simulink model "TTS2_EXT"  (R2024b)
settings: Solver=FixedStepAuto  StartTime=0.0  StopTime=inf  FixedStep=0.01  RelTol=1e-3
model workspace (MAT data in the model file):
  amp_f1 = -100
  amp_f10 = 0.5
  amp_f11 = -0.1
  amp_f12 = 1
  amp_f13 = 0.5
  amp_f14 = -20
  amp_f15 = 0.5
  amp_f16 = 0.5
  amp_f17 = 20
  amp_f18 = -30
  amp_f19 = 0.1
  amp_f2 = -20
  amp_f20 = -20
  amp_f21 = 20
  amp_f3 = -30
  amp_f4 = -30
  amp_f5 = -10
  amp_f51 = -10
  amp_f52 = -30
  amp_f53 = -30
  amp_f54 = 20
  amp_f55 = -100
  amp_f6 = -30
  amp_f7 = -30
  amp_f8 = -30
  amp_f9 = 1
  from_f1 = 570
  from_f10 = 5970
  from_f11 = 6570
  from_f12 = 7170
  from_f13 = 7770
  from_f14 = 8370
  from_f15 = 8970
  from_f16 = 9570
  from_f17 = 10170
  from_f18 = 10770
  from_f19 = 11370
  from_f2 = 1170
  from_f20 = 11970
  from_f21 = 12570
  from_f3 = 1770
  from_f4 = 2370
  from_f5 = 2970
  from_f51 = 13170
  from_f52 = 13770
  from_f53 = 14370
  from_f54 = 14970
  from_f55 = 15570
  from_f6 = 3570
  from_f7 = 4170
  from_f8 = 4770
  from_f9 = 5370
libraries: simulink x52, lab310_library x26, opclib x3
(part 2 of 3)

== system TTS2_EXT/PID/Antiwindup ==
  CV : Inport
  Logical Operator : Logic  Operator=NOR  AllPortsSameDT=off  OutDataTypeStr=boolean
  Relational Operator : RelationalOperator  Operator=<=  OutDataTypeStr=boolean  RndMeth=Simplest  InputSameDT=off
  Relational Operator1 : RelationalOperator  OutDataTypeStr=boolean  RndMeth=Simplest  InputSameDT=off
  norm CV max : Constant
  norm CVmin : Constant  Value=0
  enable : Outport  VectorParamsAs1DForOutWhenUnconnected=off
  wires:
  norm CVmin/1 -> Relational Operator/2
  norm CV max/1 -> Relational Operator1/2
  CV/1 -> Relational Operator1/1, Relational Operator/1
  Relational Operator/1 -> Logical Operator/1
  Relational Operator1/1 -> Logical Operator/2
  Logical Operator/1 -> enable/1

== system TTS2_EXT/TTS2/Disturbance ==
  Control : Inport
  Add : Sum  Inputs=2
  Add1 : Sum  Inputs=2
  Bus Selector : BusSelector  OutputSignals=PrDistValue,PrDistShift,EnPrDistShift,EnPrDist
  Product : Product
  Pulse Generator : DiscretePulseGenerator  PulseType=Time based  Period=480  PulseWidth=25
  Pulse Generator1 : DiscretePulseGenerator  PulseType=Time based  Amplitude=-1  Period=480  PulseWidth=25  PhaseDelay=240
  Switch : Switch  Criteria=u2 > Threshold  Threshold=0.5  SaturateOnIntegerOverflow=off
  Switch1 : Switch  Criteria=u2 > Threshold  Threshold=0.5  SaturateOnIntegerOverflow=off  InputSameDT=off
  no dist shift : Constant  Value=0
  dist[%] : Outport  VectorParamsAs1DForOutWhenUnconnected=off
  wires:
  Control/1 -> Bus Selector/1
  Bus Selector/2 -> Switch1/1  "<PrDistShift>"
  Bus Selector/3 -> Switch1/2  "<EnPrDistShift>"
  Switch/1 -> dist[%]/1  "PrShift+Dist"
  Switch1/1 -> Switch/3, Add/2
  Bus Selector/4 -> Switch/2  "<EnPrDist>"
  no dist shift/1 -> Switch1/3
  Add/1 -> Switch/1
  Pulse Generator/1 -> Add1/1
  Pulse Generator1/1 -> Add1/2
  Bus Selector/1 -> Product/2  "<PrDistValue>"
  Product/1 -> Add/1
  Add1/1 -> Product/1

== system TTS2_EXT/TTS2/Disturbance: Pump+pipe+control valve ==
  CV : Inport
  Patm[kPa] : Constant  Value=1.013  OutMin=[0.1013]  OutMax=[2.026]
  Pump control [%] : Constant  Value=pc  mask{pc=100.0}
      mask prompts: pc "Pump control"
  Pump+Pipe : Subsystem
  VB : Subsystem
  F[m3/h] : Outport  VectorParamsAs1DForOutWhenUnconnected=off
  wires:
  Pump+Pipe/1(P[kPa]) -> VB/2(P1[kPa])
  CV/1 -> VB/1(CV[%])
  Patm[kPa]/1 -> VB/3(P2[kPa])
  VB/1(F[m3/h]) -> Pump+Pipe/2(F[m3/h]), F[m3/h]/1
  Pump control [%]/1 -> Pump+Pipe/1(MP)

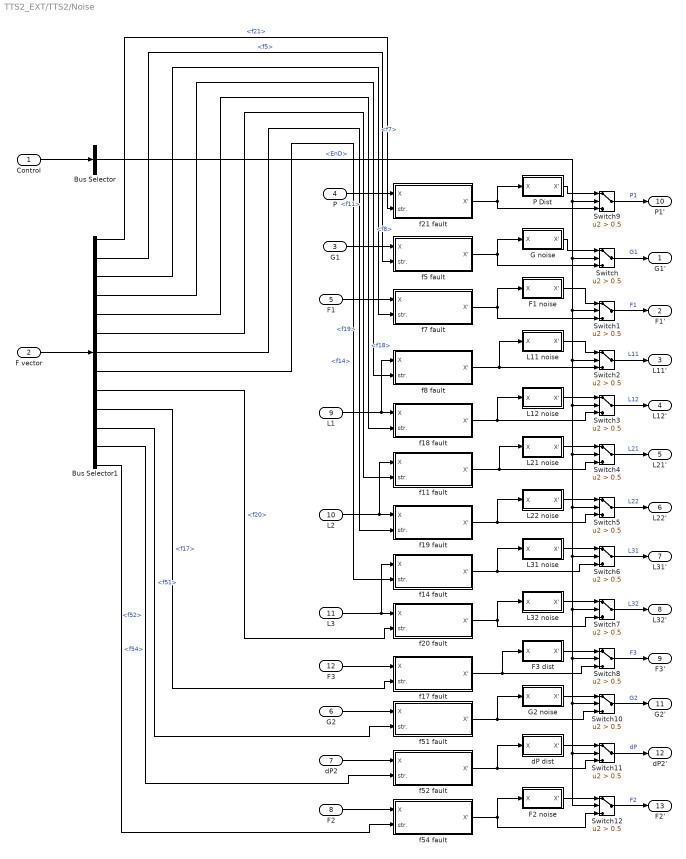
== system TTS2_EXT/TTS2/Noise ==
  Control : Inport
  F vector : Inport  Port=2
  G1 : Inport  Port=3
  P : Inport  Port=4
  F1 : Inport  Port=5
  G2 : Inport  Port=6
  dP2 : Inport  Port=7
  F2 : Inport  Port=8
  L1 : Inport  Port=9
  L2 : Inport  Port=10
  L3 : Inport  Port=11
  F3 : Inport  Port=12
  Bus Selector : BusSelector  OutputSignals=EnD
  Bus Selector1 : BusSelector  OutputSignals=f21,f5,f7,f8,f18,f11,f19,f14,f20,f17,f51,f52,f54
  F1 noise : Subsystem
  F2 noise : Subsystem
  F3 dist : Subsystem
  G noise : Subsystem
  G2 noise : Subsystem
  L11 noise : Subsystem
  L12 noise : Subsystem
  L21 noise : Subsystem
  L22 noise : Subsystem
  L31 noise : Subsystem
  L32 noise : Subsystem
  P Dist : Subsystem
  Switch{,1..12} (13 alike) : Switch  Criteria=u2 > Threshold  Threshold=0.5  SaturateOnIntegerOverflow=off  InputSameDT=off
  dP dist : Subsystem
  f11 fault : Subsystem
  f14 fault : Subsystem
  f17 fault : Subsystem
  f18 fault : Subsystem
  f19 fault : Subsystem
  f20 fault : Subsystem
  f21 fault : Subsystem
  f5 fault : Subsystem
  f51 fault : Subsystem
  f52 fault : Subsystem
  f54 fault : Subsystem
  f7 fault : Subsystem
  f8 fault : Subsystem
  G1' : Outport  VectorParamsAs1DForOutWhenUnconnected=off
  F1' : Outport  Port=2  VectorParamsAs1DForOutWhenUnconnected=off
  L11' : Outport  Port=3  VectorParamsAs1DForOutWhenUnconnected=off
  L12' : Outport  Port=4  VectorParamsAs1DForOutWhenUnconnected=off
  L21' : Outport  Port=5  VectorParamsAs1DForOutWhenUnconnected=off
  L22' : Outport  Port=6  VectorParamsAs1DForOutWhenUnconnected=off
  L31' : Outport  Port=7  VectorParamsAs1DForOutWhenUnconnected=off
  L32' : Outport  Port=8  VectorParamsAs1DForOutWhenUnconnected=off
  F3' : Outport  Port=9  VectorParamsAs1DForOutWhenUnconnected=off
  P1' : Outport  Port=10  VectorParamsAs1DForOutWhenUnconnected=off
  G2' : Outport  Port=11  VectorParamsAs1DForOutWhenUnconnected=off
  dP2' : Outport  Port=12  VectorParamsAs1DForOutWhenUnconnected=off
  F2' : Outport  Port=13  VectorParamsAs1DForOutWhenUnconnected=off
  wires:
  f21 fault/1(X') -> P Dist/1(X), Switch9/3
  P Dist/1(X') -> Switch9/1
  Switch9/1 -> P1'/1  "P1"
  P/1 -> f21 fault/1(X)
  Switch2/1 -> L11'/1  "L11"
  Switch8/1 -> F3'/1  "F3"
  Switch7/1 -> L32'/1  "L32"
  F1 noise/1(X') -> Switch1/1
  Switch3/1 -> L12'/1  "L12"
  Switch4/1 -> L21'/1  "L21"
  Switch6/1 -> L31'/1  "L31"
  L11 noise/1(X') -> Switch2/1
  G noise/1(X') -> Switch/1
  Switch5/1 -> L22'/1  "L22"
  f20 fault/1(X') -> Switch7/3, L32 noise/1(X)
  F3 dist/1(X') -> Switch8/1
  f11 fault/1(X') -> Switch4/3, L21 noise/1(X)
  L32 noise/1(X') -> Switch7/1
  L31 noise/1(X') -> Switch6/1
  f18 fault/1(X') -> Switch3/3, L12 noise/1(X)
  F1/1 -> f7 fault/1(X)
  L22 noise/1(X') -> Switch5/1
  L1/1 -> f18 fault/1(X), f8 fault/1(X)
  L2/1 -> f11 fault/1(X), f19 fault/1(X)
  Switch/1 -> G1'/1  "G1"
  f5 fault/1(X') -> Switch/3, G noise/1(X)
  L21 noise/1(X') -> Switch4/1
  f19 fault/1(X') -> Switch5/3, L22 noise/1(X)
  Bus Selector/1 -> Switch9/2, Switch8/2, Switch12/2, Switch11/2, Switch10/2, Switch7/2, Switch6/2, Switch5/2, Switch4/2, Switch3/2, Switch2/2, Switch1/2, Switch/2  "<EnD>"
  f17 fault/1(X') -> F3 dist/1(X), Switch8/3
  Switch1/1 -> F1'/1  "F1"
  L12 noise/1(X') -> Switch3/1
  f8 fault/1(X') -> Switch2/3, L11 noise/1(X)
  f14 fault/1(X') -> Switch6/3, L31 noise/1(X)
  f7 fault/1(X') -> Switch1/3, F1 noise/1(X)
  L3/1 -> f14 fault/1(X), f20 fault/1(X)
  G1/1 -> f5 fault/1(X)
  Control/1 -> Bus Selector/1
  F vector/1 -> Bus Selector1/1
  Bus Selector1/1 -> f21 fault/2(str.)  "<f21>"
  Bus Selector1/2 -> f5 fault/2(str.)  "<f5>"
  Bus Selector1/3 -> f7 fault/2(str.)  "<f7>"
  Bus Selector1/4 -> f8 fault/2(str.)  "<f8>"
  Bus Selector1/5 -> f18 fault/2(str.)  "<f18>"
  Bus Selector1/6 -> f11 fault/2(str.)  "<f11>"
  Bus Selector1/7 -> f19 fault/2(str.)  "<f19>"
  Bus Selector1/8 -> f14 fault/2(str.)  "<f14>"
  Bus Selector1/9 -> f20 fault/2(str.)  "<f20>"
  Bus Selector1/10 -> f17 fault/2(str.)  "<f17>"
  dP2/1 -> f52 fault/1(X)
  G2/1 -> f51 fault/1(X)
  Switch12/1 -> F2'/1  "F2"
  Switch11/1 -> dP2'/1  "dP"
  Switch10/1 -> G2'/1  "G2"
  f54 fault/1(X') -> F2 noise/1(X), Switch12/3
  f52 fault/1(X') -> Switch11/3, dP dist/1(X)
  f51 fault/1(X') -> Switch10/3, G2 noise/1(X)
  G2 noise/1(X') -> Switch10/1
  dP dist/1(X') -> Switch11/1
  F2 noise/1(X') -> Switch12/1
  Bus Selector1/11 -> f51 fault/2(str.)  "<f51>"
  Bus Selector1/12 -> f52 fault/2(str.)  "<f52>"
  Bus Selector1/13 -> f54 fault/2(str.)  "<f54>"
  F2/1 -> f54 fault/1(X)
  F3/1 -> f17 fault/1(X)

== system TTS2_EXT/TTS2/Pump+pipe+control valve ==
  CV1 : Inport
  F vec : Inport  Port=2
  CV2 : Inport  Port=3
  Add : Sum
  Bus Selector : BusSelector  OutputSignals=f1,f2,f4,f6,f53
  Patm[kPa] : Constant  Value=1.013  OutMin=[0.1013]  OutMax=[2.026]
  Pump control [%] : Constant  Value=pc  mask{pc=100.0}
      mask prompts: pc "Pump control"
  Pump+Pipe : Subsystem
  V1 : Subsystem
  V2 : Subsystem
  f1 fault : Subsystem
  f2 fault : Subsystem
  X1[%] : Outport  VectorParamsAs1DForOutWhenUnconnected=off
  F1[m3/s] : Outport  Port=2  VectorParamsAs1DForOutWhenUnconnected=off
  dP1[kPa] : Outport  Port=3  VectorParamsAs1DForOutWhenUnconnected=off
  P[kPa] : Outport  Port=4  VectorParamsAs1DForOutWhenUnconnected=off
  X2[%] : Outport  Port=5  VectorParamsAs1DForOutWhenUnconnected=off
  F2[m3/s] : Outport  Port=6  VectorParamsAs1DForOutWhenUnconnected=off
  dP2[kPa] : Outport  Port=7  VectorParamsAs1DForOutWhenUnconnected=off
  wires:
  Pump control [%]/1 -> f1 fault/1(X)
  f2 fault/1(Xf) -> Pump+Pipe/1(MP)
  f1 fault/1(Xf) -> f2 fault/1(X)
  Bus Selector/2 -> f2 fault/2(str.)  "<f2>"
  Bus Selector/1 -> f1 fault/2(str.)  "<f1>"
  F vec/1 -> Bus Selector/1
  Pump+Pipe/1(P[kPa]) -> P[kPa]/1, V2/2(P1[kPa]), V1/2(P1[kPa])
  CV1/1 -> V1/1(CV[%])
  Patm[kPa]/1 -> V2/3(P2[kPa]), V1/3(P2[kPa])
  Bus Selector/3 -> V1/4(f04)  "<f4>"
  Bus Selector/4 -> V1/5(f06)  "<f6>"
  V1/1(X[%]) -> X1[%]/1
  V1/3(dP[kPa]) -> dP1[kPa]/1
  V1/2(F[m3/s]) -> Add/2, F1[m3/s]/1
  CV2/1 -> V2/1(CV[%])
  V2/1(X[%]) -> X2[%]/1
  V2/2(F[m3/s]) -> Add/1, F2[m3/s]/1
  V2/3(dP[kPa]) -> dP2[kPa]/1
  Bus Selector/5 -> V2/4(f53)  "<f53>"
  Add/1 -> Pump+Pipe/2(F[m3/h])

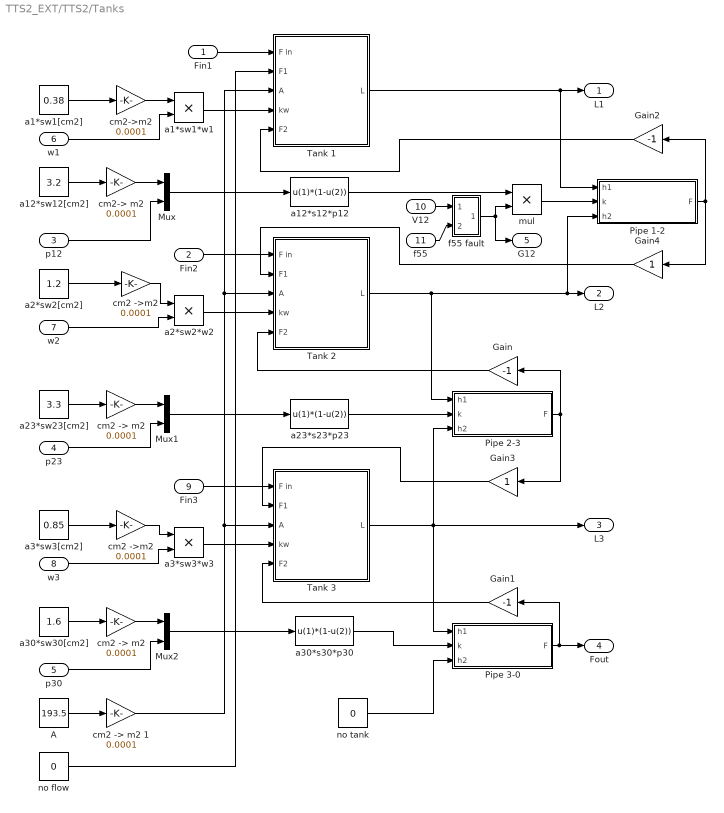
== system TTS2_EXT/TTS2/Tanks ==
  Fin1 : Inport
  Fin2 : Inport  Port=2
  p12 : Inport  Port=3
  p23 : Inport  Port=4
  p30 : Inport  Port=5
  w1 : Inport  Port=6
  w2 : Inport  Port=7
  w3 : Inport  Port=8
  Fin3 : Inport  Port=9
  V12 : Inport  Port=10
  f55 : Inport  Port=11
  A : Constant  Value=193.5
  Gain : Gain  Gain=-1
  Gain1 : Gain  Gain=-1
  Gain2 : Gain  Gain=-1
  Gain3 : Gain
  Gain4 : Gain
  Mux : Mux  Inputs=2
  Mux1 : Mux  Inputs=2
  Mux2 : Mux  Inputs=2
  Pipe 1-2 : Subsystem
  Pipe 2-3 : Subsystem
  Pipe 3-0 : Subsystem
  "Tank 1 " : Subsystem
  Tank 2 : Subsystem
  Tank 3 : Subsystem
  a1*sw1*w1 : Product
  a1*sw1[cm2] : Constant  Value=0.38
  a12*s12*p12 : Fcn  Expr=u(1)*(1-u(2))
  a12*sw12[cm2] : Constant  Value=3.2
  a2*sw2*w2 : Product
  a2*sw2[cm2] : Constant  Value=1.2
  a23*s23*p23 : Fcn  Expr=u(1)*(1-u(2))
  a23*sw23[cm2] : Constant  Value=3.3
  a3*sw3*w3 : Product
  a3*sw3[cm2] : Constant  Value=0.85
  a30*s30*p30 : Fcn  Expr=u(1)*(1-u(2))
  a30*sw30[cm2] : Constant  Value=1.6
  "cm2 -> m2" : Gain  Gain=0.0001
  "cm2 -> m2 " : Gain  Gain=0.0001
  "cm2 -> m2 1" : Gain  Gain=0.0001
  cm2 ->m2 : Gain  Gain=0.0001
  "cm2 ->m2 " : Gain  Gain=0.0001
  cm2-> m2 : Gain  Gain=0.0001
  cm2->m2 : Gain  Gain=0.0001
  f55 fault : Subsystem
  mul : Product
  no flow : Constant  Value=0
  no tank : Constant  Value=0
  L1 : Outport  VectorParamsAs1DForOutWhenUnconnected=off
  L2 : Outport  Port=2  VectorParamsAs1DForOutWhenUnconnected=off
  L3 : Outport  Port=3  VectorParamsAs1DForOutWhenUnconnected=off
  Fout : Outport  Port=4  VectorParamsAs1DForOutWhenUnconnected=off
  G12 : Outport  Port=5  VectorParamsAs1DForOutWhenUnconnected=off
  wires:
  Fin1/1 -> "Tank 1 "/1(F in)
  a1*sw1[cm2]/1 -> cm2->m2/1
  cm2->m2/1 -> a1*sw1*w1/1
  a1*sw1*w1/1 -> "Tank 1 "/4(kw)
  w1/1 -> a1*sw1*w1/2
  a12*sw12[cm2]/1 -> cm2-> m2/1
  cm2-> m2/1 -> Mux/1
  p12/1 -> Mux/2
  Mux/1 -> a12*s12*p12/1
  a2*sw2[cm2]/1 -> cm2 ->m2/1
  cm2 ->m2/1 -> a2*sw2*w2/1
  a23*sw23[cm2]/1 -> "cm2 -> m2"/1
  "cm2 -> m2"/1 -> Mux1/1
  Mux1/1 -> a23*s23*p23/1
  w2/1 -> a2*sw2*w2/2
  p23/1 -> Mux1/2
  a2*sw2*w2/1 -> Tank 2/4(kw)
  a3*sw3[cm2]/1 -> "cm2 ->m2 "/1
  "cm2 ->m2 "/1 -> a3*sw3*w3/1
  a30*sw30[cm2]/1 -> "cm2 -> m2 "/1
  "cm2 -> m2 "/1 -> Mux2/1
  w3/1 -> a3*sw3*w3/2
  p30/1 -> Mux2/2
  Mux2/1 -> a30*s30*p30/1
  a3*sw3*w3/1 -> Tank 3/4(kw)
  A/1 -> "cm2 -> m2 1"/1
  no flow/1 -> "Tank 1 "/2(F1)
  "cm2 -> m2 1"/1 -> Tank 3/3(A), Tank 2/3(A), "Tank 1 "/3(A)
  "Tank 1 "/1(L) -> Pipe 1-2/1(h1), L1/1
  a12*s12*p12/1 -> mul/1
  Tank 2/1(L) -> Pipe 1-2/3(h2), L2/1, Pipe 2-3/1(h1)
  a23*s23*p23/1 -> Pipe 2-3/2(k)
  Tank 3/1(L) -> Pipe 2-3/3(h2), Pipe 3-0/1(h1), L3/1
  a30*s30*p30/1 -> Pipe 3-0/2(k)
  no tank/1 -> Pipe 3-0/3(h2)
  Pipe 3-0/1(F) -> Fout/1, Gain1/1
  Pipe 2-3/1(F) -> Gain3/1, Gain/1
  Pipe 1-2/1(F) -> Gain2/1, Gain4/1
  Gain2/1 -> "Tank 1 "/5(F2)
  Gain/1 -> Tank 2/5(F2)
  Fin3/1 -> Tank 3/1(F in)
  Gain1/1 -> Tank 3/5(F2)
  Gain3/1 -> Tank 3/2(F1)
  Gain4/1 -> Tank 2/2(F1)
  Fin2/1 -> Tank 2/1(F in)
  mul/1 -> Pipe 1-2/2(k)
  V12/1 -> f55 fault/1(X)
  f55/1 -> f55 fault/2(str.)
  f55 fault/1(X') -> G12/1, mul/2

== system TTS2_EXT/TTS2/f3 fault ==
  X : Inport
  str. : Inport  Port=2
  Add : Sum
  Fcn : Fcn  Expr=u(1)*((u(2)/100)+1)
  Manual Switch : ManualSwitch  CurrentSetting=0
  Mux : Mux  Inputs=2
  X' : Outport  VectorParamsAs1DForOutWhenUnconnected=off
  wires:
  Mux/1 -> Fcn/1
  X/1 -> Add/1, Mux/1
  str./1 -> Add/2, Mux/2
  Manual Switch/1 -> X'/1
  Add/1 -> Manual Switch/1
  Fcn/1 -> Manual Switch/2

== system TTS2_EXT/Faults/f-control1/calc_f1 ==
  f-control : Inport
  f-s : Inport  Port=2
  Bus Selector : BusSelector  OutputSignals=EnF,AutoF
  Bus Selector1 : BusSelector  OutputSignals=f1
  Constant : Constant  Value=p
  Product : Product  Inputs=3
  Step : Step  Time=from  After=amp  SampleTime=0
  Step1 : Step  Time=from+st  After=-amp  SampleTime=0
  Subsystem : Subsystem
  Sum1 : Sum  Inputs=++|
  Switch:auto : Switch  Criteria=u2 > Threshold  Threshold=0.5  SaturateOnIntegerOverflow=off  InputSameDT=off
  f : Outport  VectorParamsAs1DForOutWhenUnconnected=off
  wires:
  f-control/1 -> Bus Selector/1
  f-s/1 -> Bus Selector1/1
  Product/1 -> f/1
  Bus Selector/1 -> Product/1  "<EnF>"
  Bus Selector/2 -> Switch:auto/2  "<AutoF>"
  Switch:auto/1 -> Product/2
  Step/1 -> Sum1/2
  Step1/1 -> Sum1/1
  Constant/1 -> Product/3
  Bus Selector1/1 -> Subsystem/1(w)  "<f1>"
  Subsystem/1(w_sim) -> Switch:auto/3
  Sum1/1 -> Switch:auto/1

== system TTS2_EXT/Faults/f-control1/calc_f10 ==
  f-control : Inport
  f-s : Inport  Port=2
  Bus Selector : BusSelector  OutputSignals=EnF,IncipF,AutoF
  Bus Selector1 : BusSelector  OutputSignals=f10
  Constant : Constant  Value=p
  Product : Product  Inputs=3
  RAMP : simulink/Sources/Ramp  slope=amp/st  start=from  InitialOutput=0
  Saturation : Saturate  UpperLimit=abs(amp)  LowerLimit=-abs(amp)
  Step : Step  Time=from  After=amp  SampleTime=0
  Step1 : Step  Time=from+st  After=-amp  SampleTime=0
  Subsystem : Subsystem
  Sum : Sum  Inputs=|++
  Sum1 : Sum  Inputs=++|
  Switch:auto : Switch  Criteria=u2 > Threshold  Threshold=0.5  SaturateOnIntegerOverflow=off  InputSameDT=off
  Switch:kind : Switch  Criteria=u2 > Threshold  Threshold=0.5  SaturateOnIntegerOverflow=off  InputSameDT=off
  f : Outport  VectorParamsAs1DForOutWhenUnconnected=off
  wires:
  f-control/1 -> Bus Selector/1
  f-s/1 -> Bus Selector1/1
  Product/1 -> f/1
  Bus Selector/1 -> Product/1  "<EnF>"
  Bus Selector/2 -> Subsystem/1(IncipF), Switch:kind/2  "<IncipF>"
  Bus Selector/3 -> Switch:auto/2  "<AutoF>"
  Switch:auto/1 -> Product/2
  Sum/1 -> Switch:kind/1
  Sum1/1 -> Switch:kind/3
  Switch:kind/1 -> Switch:auto/1
  Step/1 -> Sum1/2
  Step1/1 -> Sum/2, Sum1/1
  Saturation/1 -> Sum/1
  RAMP/1 -> Saturation/1
  Constant/1 -> Product/3
  Bus Selector1/1 -> Subsystem/2(w)  "<f10>"
  Subsystem/1(w_sim) -> Switch:auto/3

== system TTS2_EXT/Faults/f-control1/calc_f11 ==
  f-control : Inport
  f-s : Inport  Port=2
  Bus Selector : BusSelector  OutputSignals=EnF,IncipF,AutoF
  Bus Selector1 : BusSelector  OutputSignals=f11
  Constant : Constant  Value=p
  Product : Product  Inputs=3
  RAMP : simulink/Sources/Ramp  slope=amp/st  start=from  InitialOutput=0
  Saturation : Saturate  UpperLimit=abs(amp)  LowerLimit=-abs(amp)
  Step : Step  Time=from  After=amp  SampleTime=0
  Step1 : Step  Time=from+st  After=-amp  SampleTime=0
  Subsystem : Subsystem
  Sum : Sum  Inputs=|++
  Sum1 : Sum  Inputs=++|
  Switch:auto : Switch  Criteria=u2 > Threshold  Threshold=0.5  SaturateOnIntegerOverflow=off  InputSameDT=off
  Switch:kind : Switch  Criteria=u2 > Threshold  Threshold=0.5  SaturateOnIntegerOverflow=off  InputSameDT=off
  f : Outport  VectorParamsAs1DForOutWhenUnconnected=off
  wires:
  f-control/1 -> Bus Selector/1
  f-s/1 -> Bus Selector1/1
  Product/1 -> f/1
  Bus Selector/1 -> Product/1  "<EnF>"
  Bus Selector/2 -> Subsystem/1(IncipF), Switch:kind/2  "<IncipF>"
  Bus Selector/3 -> Switch:auto/2  "<AutoF>"
  Switch:auto/1 -> Product/2
  Sum/1 -> Switch:kind/1
  Sum1/1 -> Switch:kind/3
  Switch:kind/1 -> Switch:auto/1
  Step/1 -> Sum1/2
  Step1/1 -> Sum/2, Sum1/1
  Saturation/1 -> Sum/1
  RAMP/1 -> Saturation/1
  Constant/1 -> Product/3
  Bus Selector1/1 -> Subsystem/2(w)  "<f11>"
  Subsystem/1(w_sim) -> Switch:auto/3

== system TTS2_EXT/Faults/f-control1/calc_f12 ==
  f-control : Inport
  f-s : Inport  Port=2
  Bus Selector : BusSelector  OutputSignals=EnF,IncipF,AutoF
  Bus Selector1 : BusSelector  OutputSignals=f12
  Constant : Constant  Value=p
  Product : Product  Inputs=3
  RAMP : simulink/Sources/Ramp  slope=amp/st  start=from  InitialOutput=0
  Saturation : Saturate  UpperLimit=abs(amp)  LowerLimit=-abs(amp)
  Step : Step  Time=from  After=amp  SampleTime=0
  Step1 : Step  Time=from+st  After=-amp  SampleTime=0
  Subsystem : Subsystem
  Sum : Sum  Inputs=|++
  Sum1 : Sum  Inputs=++|
  Switch:auto : Switch  Criteria=u2 > Threshold  Threshold=0.5  SaturateOnIntegerOverflow=off  InputSameDT=off
  Switch:kind : Switch  Criteria=u2 > Threshold  Threshold=0.5  SaturateOnIntegerOverflow=off  InputSameDT=off
  f : Outport  VectorParamsAs1DForOutWhenUnconnected=off
  wires:
  f-control/1 -> Bus Selector/1
  f-s/1 -> Bus Selector1/1
  Product/1 -> f/1
  Bus Selector/1 -> Product/1  "<EnF>"
  Bus Selector/2 -> Subsystem/1(IncipF), Switch:kind/2  "<IncipF>"
  Bus Selector/3 -> Switch:auto/2  "<AutoF>"
  Switch:auto/1 -> Product/2
  Sum/1 -> Switch:kind/1
  Sum1/1 -> Switch:kind/3
  Switch:kind/1 -> Switch:auto/1
  Step/1 -> Sum1/2
  Step1/1 -> Sum/2, Sum1/1
  Saturation/1 -> Sum/1
  RAMP/1 -> Saturation/1
  Constant/1 -> Product/3
  Bus Selector1/1 -> Subsystem/2(w)  "<f12>"
  Subsystem/1(w_sim) -> Switch:auto/3

== system TTS2_EXT/Faults/f-control1/calc_f13 ==
  f-control : Inport
  f-s : Inport  Port=2
  Bus Selector : BusSelector  OutputSignals=EnF,IncipF,AutoF
  Bus Selector1 : BusSelector  OutputSignals=f13
  Constant : Constant  Value=p
  Product : Product  Inputs=3
  RAMP : simulink/Sources/Ramp  slope=amp/st  start=from  InitialOutput=0
  Saturation : Saturate  UpperLimit=abs(amp)  LowerLimit=-abs(amp)
  Step : Step  Time=from  After=amp  SampleTime=0
  Step1 : Step  Time=from+st  After=-amp  SampleTime=0
  Subsystem : Subsystem
  Sum : Sum  Inputs=|++
  Sum1 : Sum  Inputs=++|
  Switch:auto : Switch  Criteria=u2 > Threshold  Threshold=0.5  SaturateOnIntegerOverflow=off  InputSameDT=off
  Switch:kind : Switch  Criteria=u2 > Threshold  Threshold=0.5  SaturateOnIntegerOverflow=off  InputSameDT=off
  f : Outport  VectorParamsAs1DForOutWhenUnconnected=off
  wires:
  f-control/1 -> Bus Selector/1
  f-s/1 -> Bus Selector1/1
  Product/1 -> f/1
  Bus Selector/1 -> Product/1  "<EnF>"
  Bus Selector/2 -> Subsystem/1(IncipF), Switch:kind/2  "<IncipF>"
  Bus Selector/3 -> Switch:auto/2  "<AutoF>"
  Switch:auto/1 -> Product/2
  Sum/1 -> Switch:kind/1
  Sum1/1 -> Switch:kind/3
  Switch:kind/1 -> Switch:auto/1
  Step/1 -> Sum1/2
  Step1/1 -> Sum/2, Sum1/1
  Saturation/1 -> Sum/1
  RAMP/1 -> Saturation/1
  Constant/1 -> Product/3
  Bus Selector1/1 -> Subsystem/2(w)  "<f13>"
  Subsystem/1(w_sim) -> Switch:auto/3

== system TTS2_EXT/Faults/f-control1/calc_f14 ==
  f-control : Inport
  f-s : Inport  Port=2
  Bus Selector : BusSelector  OutputSignals=EnF,IncipF,AutoF
  Bus Selector1 : BusSelector  OutputSignals=f14
  Constant : Constant  Value=p
  Product : Product  Inputs=3
  RAMP : simulink/Sources/Ramp  slope=amp/st  start=from  InitialOutput=0
  Saturation : Saturate  UpperLimit=abs(amp)  LowerLimit=-abs(amp)
  Step : Step  Time=from  After=amp  SampleTime=0
  Step1 : Step  Time=from+st  After=-amp  SampleTime=0
  Subsystem : Subsystem
  Sum : Sum  Inputs=|++
  Sum1 : Sum  Inputs=++|
  Switch:auto : Switch  Criteria=u2 > Threshold  Threshold=0.5  SaturateOnIntegerOverflow=off  InputSameDT=off
  Switch:kind : Switch  Criteria=u2 > Threshold  Threshold=0.5  SaturateOnIntegerOverflow=off  InputSameDT=off
  f : Outport  VectorParamsAs1DForOutWhenUnconnected=off
  wires:
  f-control/1 -> Bus Selector/1
  f-s/1 -> Bus Selector1/1
  Product/1 -> f/1
  Bus Selector/1 -> Product/1  "<EnF>"
  Bus Selector/2 -> Subsystem/1(IncipF), Switch:kind/2  "<IncipF>"
  Bus Selector/3 -> Switch:auto/2  "<AutoF>"
  Switch:auto/1 -> Product/2
  Sum/1 -> Switch:kind/1
  Sum1/1 -> Switch:kind/3
  Switch:kind/1 -> Switch:auto/1
  Step/1 -> Sum1/2
  Step1/1 -> Sum/2, Sum1/1
  Saturation/1 -> Sum/1
  RAMP/1 -> Saturation/1
  Constant/1 -> Product/3
  Bus Selector1/1 -> Subsystem/2(w)  "<f14>"
  Subsystem/1(w_sim) -> Switch:auto/3

== system TTS2_EXT/Faults/f-control1/calc_f15 ==
  f-control : Inport
  f-s : Inport  Port=2
  Bus Selector : BusSelector  OutputSignals=EnF,IncipF,AutoF
  Bus Selector1 : BusSelector  OutputSignals=f15
  Constant : Constant  Value=p
  Product : Product  Inputs=3
  RAMP : simulink/Sources/Ramp  slope=amp/st  start=from  InitialOutput=0
  Saturation : Saturate  UpperLimit=abs(amp)  LowerLimit=-abs(amp)
  Step : Step  Time=from  After=amp  SampleTime=0
  Step1 : Step  Time=from+st  After=-amp  SampleTime=0
  Subsystem : Subsystem
  Sum : Sum  Inputs=|++
  Sum1 : Sum  Inputs=++|
  Switch:auto : Switch  Criteria=u2 > Threshold  Threshold=0.5  SaturateOnIntegerOverflow=off  InputSameDT=off
  Switch:kind : Switch  Criteria=u2 > Threshold  Threshold=0.5  SaturateOnIntegerOverflow=off  InputSameDT=off
  f : Outport  VectorParamsAs1DForOutWhenUnconnected=off
  wires:
  f-control/1 -> Bus Selector/1
  f-s/1 -> Bus Selector1/1
  Product/1 -> f/1
  Bus Selector/1 -> Product/1  "<EnF>"
  Bus Selector/2 -> Subsystem/1(IncipF), Switch:kind/2  "<IncipF>"
  Bus Selector/3 -> Switch:auto/2  "<AutoF>"
  Switch:auto/1 -> Product/2
  Sum/1 -> Switch:kind/1
  Sum1/1 -> Switch:kind/3
  Switch:kind/1 -> Switch:auto/1
  Step/1 -> Sum1/2
  Step1/1 -> Sum/2, Sum1/1
  Saturation/1 -> Sum/1
  RAMP/1 -> Saturation/1
  Constant/1 -> Product/3
  Bus Selector1/1 -> Subsystem/2(w)  "<f15>"
  Subsystem/1(w_sim) -> Switch:auto/3

== system TTS2_EXT/Faults/f-control1/calc_f16 ==
  f-control : Inport
  f-s : Inport  Port=2
  Bus Selector : BusSelector  OutputSignals=EnF,IncipF,AutoF
  Bus Selector1 : BusSelector  OutputSignals=f16
  Constant : Constant  Value=p
  Product : Product  Inputs=3
  RAMP : simulink/Sources/Ramp  slope=amp/st  start=from  InitialOutput=0
  Saturation : Saturate  UpperLimit=abs(amp)  LowerLimit=-abs(amp)
  Step : Step  Time=from  After=amp  SampleTime=0
  Step1 : Step  Time=from+st  After=-amp  SampleTime=0
  Subsystem : Subsystem
  Sum : Sum  Inputs=|++
  Sum1 : Sum  Inputs=++|
  Switch:auto : Switch  Criteria=u2 > Threshold  Threshold=0.5  SaturateOnIntegerOverflow=off  InputSameDT=off
  Switch:kind : Switch  Criteria=u2 > Threshold  Threshold=0.5  SaturateOnIntegerOverflow=off  InputSameDT=off
  f : Outport  VectorParamsAs1DForOutWhenUnconnected=off
  wires:
  f-control/1 -> Bus Selector/1
  f-s/1 -> Bus Selector1/1
  Product/1 -> f/1
  Bus Selector/1 -> Product/1  "<EnF>"
  Bus Selector/2 -> Subsystem/1(IncipF), Switch:kind/2  "<IncipF>"
  Bus Selector/3 -> Switch:auto/2  "<AutoF>"
  Switch:auto/1 -> Product/2
  Sum/1 -> Switch:kind/1
  Sum1/1 -> Switch:kind/3
  Switch:kind/1 -> Switch:auto/1
  Step/1 -> Sum1/2
  Step1/1 -> Sum/2, Sum1/1
  Saturation/1 -> Sum/1
  RAMP/1 -> Saturation/1
  Constant/1 -> Product/3
  Bus Selector1/1 -> Subsystem/2(w)  "<f16>"
  Subsystem/1(w_sim) -> Switch:auto/3

== system TTS2_EXT/Faults/f-control1/calc_f17 ==
  f-control : Inport
  f-s : Inport  Port=2
  Bus Selector : BusSelector  OutputSignals=EnF,IncipF,AutoF
  Bus Selector1 : BusSelector  OutputSignals=f17
  Constant : Constant  Value=p
  Product : Product  Inputs=3
  RAMP : simulink/Sources/Ramp  slope=amp/st  start=from  InitialOutput=0
  Saturation : Saturate  UpperLimit=abs(amp)  LowerLimit=-abs(amp)
  Step : Step  Time=from  After=amp  SampleTime=0
  Step1 : Step  Time=from+st  After=-amp  SampleTime=0
  Subsystem : Subsystem
  Sum : Sum  Inputs=|++
  Sum1 : Sum  Inputs=++|
  Switch:auto : Switch  Criteria=u2 > Threshold  Threshold=0.5  SaturateOnIntegerOverflow=off  InputSameDT=off
  Switch:kind : Switch  Criteria=u2 > Threshold  Threshold=0.5  SaturateOnIntegerOverflow=off  InputSameDT=off
  f : Outport  VectorParamsAs1DForOutWhenUnconnected=off
  wires:
  f-control/1 -> Bus Selector/1
  f-s/1 -> Bus Selector1/1
  Product/1 -> f/1
  Bus Selector/1 -> Product/1  "<EnF>"
  Bus Selector/2 -> Subsystem/1(IncipF), Switch:kind/2  "<IncipF>"
  Bus Selector/3 -> Switch:auto/2  "<AutoF>"
  Switch:auto/1 -> Product/2
  Sum/1 -> Switch:kind/1
  Sum1/1 -> Switch:kind/3
  Switch:kind/1 -> Switch:auto/1
  Step/1 -> Sum1/2
  Step1/1 -> Sum/2, Sum1/1
  Saturation/1 -> Sum/1
  RAMP/1 -> Saturation/1
  Constant/1 -> Product/3
  Bus Selector1/1 -> Subsystem/2(w)  "<f17>"
  Subsystem/1(w_sim) -> Switch:auto/3

== system TTS2_EXT/Faults/f-control1/calc_f18 ==
  f-control : Inport
  f-s : Inport  Port=2
  Bus Selector : BusSelector  OutputSignals=EnF,IncipF,AutoF
  Bus Selector1 : BusSelector  OutputSignals=f18
  Constant : Constant  Value=p
  Product : Product  Inputs=3
  RAMP : simulink/Sources/Ramp  slope=amp/st  start=from  InitialOutput=0
  Saturation : Saturate  UpperLimit=abs(amp)  LowerLimit=-abs(amp)
  Step : Step  Time=from  After=amp  SampleTime=0
  Step1 : Step  Time=from+st  After=-amp  SampleTime=0
  Subsystem : Subsystem
  Sum : Sum  Inputs=|++
  Sum1 : Sum  Inputs=++|
  Switch:auto : Switch  Criteria=u2 > Threshold  Threshold=0.5  SaturateOnIntegerOverflow=off  InputSameDT=off
  Switch:kind : Switch  Criteria=u2 > Threshold  Threshold=0.5  SaturateOnIntegerOverflow=off  InputSameDT=off
  f : Outport  VectorParamsAs1DForOutWhenUnconnected=off
  wires:
  f-control/1 -> Bus Selector/1
  f-s/1 -> Bus Selector1/1
  Product/1 -> f/1
  Bus Selector/1 -> Product/1  "<EnF>"
  Bus Selector/2 -> Subsystem/1(IncipF), Switch:kind/2  "<IncipF>"
  Bus Selector/3 -> Switch:auto/2  "<AutoF>"
  Switch:auto/1 -> Product/2
  Sum/1 -> Switch:kind/1
  Sum1/1 -> Switch:kind/3
  Switch:kind/1 -> Switch:auto/1
  Step/1 -> Sum1/2
  Step1/1 -> Sum/2, Sum1/1
  Saturation/1 -> Sum/1
  RAMP/1 -> Saturation/1
  Constant/1 -> Product/3
  Bus Selector1/1 -> Subsystem/2(w)  "<f18>"
  Subsystem/1(w_sim) -> Switch:auto/3

== system TTS2_EXT/Faults/f-control1/calc_f19 ==
  f-control : Inport
  f-s : Inport  Port=2
  Bus Selector : BusSelector  OutputSignals=EnF,IncipF,AutoF
  Bus Selector1 : BusSelector  OutputSignals=f19
  Constant : Constant  Value=p
  Product : Product  Inputs=3
  RAMP : simulink/Sources/Ramp  slope=amp/st  start=from  InitialOutput=0
  Saturation : Saturate  UpperLimit=abs(amp)  LowerLimit=-abs(amp)
  Step : Step  Time=from  After=amp  SampleTime=0
  Step1 : Step  Time=from+st  After=-amp  SampleTime=0
  Subsystem : Subsystem
  Sum : Sum  Inputs=|++
  Sum1 : Sum  Inputs=++|
  Switch:auto : Switch  Criteria=u2 > Threshold  Threshold=0.5  SaturateOnIntegerOverflow=off  InputSameDT=off
  Switch:kind : Switch  Criteria=u2 > Threshold  Threshold=0.5  SaturateOnIntegerOverflow=off  InputSameDT=off
  f : Outport  VectorParamsAs1DForOutWhenUnconnected=off
  wires:
  f-control/1 -> Bus Selector/1
  f-s/1 -> Bus Selector1/1
  Product/1 -> f/1
  Bus Selector/1 -> Product/1  "<EnF>"
  Bus Selector/2 -> Subsystem/1(IncipF), Switch:kind/2  "<IncipF>"
  Bus Selector/3 -> Switch:auto/2  "<AutoF>"
  Switch:auto/1 -> Product/2
  Sum/1 -> Switch:kind/1
  Sum1/1 -> Switch:kind/3
  Switch:kind/1 -> Switch:auto/1
  Step/1 -> Sum1/2
  Step1/1 -> Sum/2, Sum1/1
  Saturation/1 -> Sum/1
  RAMP/1 -> Saturation/1
  Constant/1 -> Product/3
  Bus Selector1/1 -> Subsystem/2(w)  "<f19>"
  Subsystem/1(w_sim) -> Switch:auto/3

== system TTS2_EXT/Faults/f-control1/calc_f2 ==
  f-control : Inport
  f-s : Inport  Port=2
  Bus Selector : BusSelector  OutputSignals=EnF,IncipF,AutoF
  Bus Selector1 : BusSelector  OutputSignals=f2
  Constant : Constant  Value=p
  Product : Product  Inputs=3
  RAMP : simulink/Sources/Ramp  slope=amp/st  start=from  InitialOutput=0
  Saturation : Saturate  UpperLimit=abs(amp)  LowerLimit=-abs(amp)
  Step : Step  Time=from  After=amp  SampleTime=0
  Step1 : Step  Time=from+st  After=-amp  SampleTime=0
  Subsystem : Subsystem
  Sum : Sum  Inputs=|++
  Sum1 : Sum  Inputs=++|
  Switch:auto : Switch  Criteria=u2 > Threshold  Threshold=0.5  SaturateOnIntegerOverflow=off  InputSameDT=off
  Switch:kind : Switch  Criteria=u2 > Threshold  Threshold=0.5  SaturateOnIntegerOverflow=off  InputSameDT=off
  f : Outport  VectorParamsAs1DForOutWhenUnconnected=off
  wires:
  f-control/1 -> Bus Selector/1
  f-s/1 -> Bus Selector1/1
  Product/1 -> f/1
  Bus Selector/1 -> Product/1  "<EnF>"
  Bus Selector/2 -> Subsystem/1(IncipF), Switch:kind/2  "<IncipF>"
  Bus Selector/3 -> Switch:auto/2  "<AutoF>"
  Switch:auto/1 -> Product/2
  Sum/1 -> Switch:kind/1
  Sum1/1 -> Switch:kind/3
  Switch:kind/1 -> Switch:auto/1
  Step/1 -> Sum1/2
  Step1/1 -> Sum/2, Sum1/1
  Saturation/1 -> Sum/1
  RAMP/1 -> Saturation/1
  Constant/1 -> Product/3
  Subsystem/1(w_sim) -> Switch:auto/3
  Bus Selector1/1 -> Subsystem/2(w)  "<f2>"

== system TTS2_EXT/Faults/f-control1/calc_f20 ==
  f-control : Inport
  f-s : Inport  Port=2
  Bus Selector : BusSelector  OutputSignals=EnF,IncipF,AutoF
  Bus Selector1 : BusSelector  OutputSignals=f20
  Constant : Constant  Value=p
  Product : Product  Inputs=3
  RAMP : simulink/Sources/Ramp  slope=amp/st  start=from  InitialOutput=0
  Saturation : Saturate  UpperLimit=abs(amp)  LowerLimit=-abs(amp)
  Step : Step  Time=from  After=amp  SampleTime=0
  Step1 : Step  Time=from+st  After=-amp  SampleTime=0
  Subsystem : Subsystem
  Sum : Sum  Inputs=|++
  Sum1 : Sum  Inputs=++|
  Switch:auto : Switch  Criteria=u2 > Threshold  Threshold=0.5  SaturateOnIntegerOverflow=off  InputSameDT=off
  Switch:kind : Switch  Criteria=u2 > Threshold  Threshold=0.5  SaturateOnIntegerOverflow=off  InputSameDT=off
  f : Outport  VectorParamsAs1DForOutWhenUnconnected=off
  wires:
  f-control/1 -> Bus Selector/1
  f-s/1 -> Bus Selector1/1
  Product/1 -> f/1
  Bus Selector/1 -> Product/1  "<EnF>"
  Bus Selector/2 -> Subsystem/1(IncipF), Switch:kind/2  "<IncipF>"
  Bus Selector/3 -> Switch:auto/2  "<AutoF>"
  Switch:auto/1 -> Product/2
  Sum/1 -> Switch:kind/1
  Sum1/1 -> Switch:kind/3
  Switch:kind/1 -> Switch:auto/1
  Step/1 -> Sum1/2
  Step1/1 -> Sum/2, Sum1/1
  Saturation/1 -> Sum/1
  RAMP/1 -> Saturation/1
  Constant/1 -> Product/3
  Bus Selector1/1 -> Subsystem/2(w)  "<f20>"
  Subsystem/1(w_sim) -> Switch:auto/3

== system TTS2_EXT/Faults/f-control1/calc_f21 ==
  f-control : Inport
  f-s : Inport  Port=2
  Bus Selector : BusSelector  OutputSignals=EnF,IncipF,AutoF
  Bus Selector1 : BusSelector  OutputSignals=f21
  Constant : Constant  Value=p
  Product : Product  Inputs=3
  RAMP : simulink/Sources/Ramp  slope=amp/st  start=from  InitialOutput=0
  Saturation : Saturate  UpperLimit=abs(amp)  LowerLimit=-abs(amp)
  Step : Step  Time=from  After=amp  SampleTime=0
  Step1 : Step  Time=from+st  After=-amp  SampleTime=0
  Subsystem : Subsystem
  Sum : Sum  Inputs=|++
  Sum1 : Sum  Inputs=++|
  Switch:auto : Switch  Criteria=u2 > Threshold  Threshold=0.5  SaturateOnIntegerOverflow=off  InputSameDT=off
  Switch:kind : Switch  Criteria=u2 > Threshold  Threshold=0.5  SaturateOnIntegerOverflow=off  InputSameDT=off
  f : Outport  VectorParamsAs1DForOutWhenUnconnected=off
  wires:
  f-control/1 -> Bus Selector/1
  f-s/1 -> Bus Selector1/1
  Product/1 -> f/1
  Bus Selector/1 -> Product/1  "<EnF>"
  Bus Selector/2 -> Subsystem/1(IncipF), Switch:kind/2  "<IncipF>"
  Bus Selector/3 -> Switch:auto/2  "<AutoF>"
  Switch:auto/1 -> Product/2
  Sum/1 -> Switch:kind/1
  Sum1/1 -> Switch:kind/3
  Switch:kind/1 -> Switch:auto/1
  Step/1 -> Sum1/2
  Step1/1 -> Sum/2, Sum1/1
  Saturation/1 -> Sum/1
  RAMP/1 -> Saturation/1
  Constant/1 -> Product/3
  Bus Selector1/1 -> Subsystem/2(w)  "<f21>"
  Subsystem/1(w_sim) -> Switch:auto/3

== system TTS2_EXT/Faults/f-control1/calc_f22 ==
  f-control : Inport
  f-s : Inport  Port=2
  Bus Selector : BusSelector  OutputSignals=EnF,IncipF,AutoF
  Bus Selector1 : BusSelector  OutputSignals=f4
  Constant : Constant  Value=p
  Product : Product  Inputs=3
  RAMP : simulink/Sources/Ramp  slope=amp/st  start=from  InitialOutput=0
  Saturation : Saturate  UpperLimit=abs(amp)  LowerLimit=-abs(amp)
  Step : Step  Time=from  After=amp  SampleTime=0
  Step1 : Step  Time=from+st  After=-amp  SampleTime=0
  Subsystem : Subsystem
  Sum : Sum  Inputs=|++
  Sum1 : Sum  Inputs=++|
  Switch:auto : Switch  Criteria=u2 > Threshold  Threshold=0.5  SaturateOnIntegerOverflow=off  InputSameDT=off
  Switch:kind : Switch  Criteria=u2 > Threshold  Threshold=0.5  SaturateOnIntegerOverflow=off  InputSameDT=off
  f : Outport  VectorParamsAs1DForOutWhenUnconnected=off
  wires:
  f-control/1 -> Bus Selector/1
  f-s/1 -> Bus Selector1/1
  Product/1 -> f/1
  Bus Selector/1 -> Product/1  "<EnF>"
  Bus Selector/2 -> Subsystem/1(IncipF), Switch:kind/2  "<IncipF>"
  Bus Selector/3 -> Switch:auto/2  "<AutoF>"
  Switch:auto/1 -> Product/2
  Sum/1 -> Switch:kind/1
  Sum1/1 -> Switch:kind/3
  Switch:kind/1 -> Switch:auto/1
  Step/1 -> Sum1/2
  Step1/1 -> Sum/2, Sum1/1
  Saturation/1 -> Sum/1
  RAMP/1 -> Saturation/1
  Constant/1 -> Product/3
  Bus Selector1/1 -> Subsystem/2(w)  "<f4>"
  Subsystem/1(w_sim) -> Switch:auto/3

== system TTS2_EXT/Faults/f-control1/calc_f4 ==
  f-control : Inport
  f-s : Inport  Port=2
  Bus Selector : BusSelector  OutputSignals=EnF,IncipF,AutoF
  Bus Selector1 : BusSelector  OutputSignals=f4
  Constant : Constant  Value=p
  Product : Product  Inputs=3
  RAMP : simulink/Sources/Ramp  slope=amp/st  start=from  InitialOutput=0
  Saturation : Saturate  UpperLimit=abs(amp)  LowerLimit=-abs(amp)
  Step : Step  Time=from  After=amp  SampleTime=0
  Step1 : Step  Time=from+st  After=-amp  SampleTime=0
  Subsystem : Subsystem
  Sum : Sum  Inputs=|++
  Sum1 : Sum  Inputs=++|
  Switch:auto : Switch  Criteria=u2 > Threshold  Threshold=0.5  SaturateOnIntegerOverflow=off  InputSameDT=off
  Switch:kind : Switch  Criteria=u2 > Threshold  Threshold=0.5  SaturateOnIntegerOverflow=off  InputSameDT=off
  f : Outport  VectorParamsAs1DForOutWhenUnconnected=off
  wires:
  f-control/1 -> Bus Selector/1
  f-s/1 -> Bus Selector1/1
  Product/1 -> f/1
  Bus Selector/1 -> Product/1  "<EnF>"
  Bus Selector/2 -> Subsystem/1(IncipF), Switch:kind/2  "<IncipF>"
  Bus Selector/3 -> Switch:auto/2  "<AutoF>"
  Switch:auto/1 -> Product/2
  Sum/1 -> Switch:kind/1
  Sum1/1 -> Switch:kind/3
  Switch:kind/1 -> Switch:auto/1
  Step/1 -> Sum1/2
  Step1/1 -> Sum/2, Sum1/1
  Saturation/1 -> Sum/1
  RAMP/1 -> Saturation/1
  Constant/1 -> Product/3
  Bus Selector1/1 -> Subsystem/2(w)  "<f4>"
  Subsystem/1(w_sim) -> Switch:auto/3

== system TTS2_EXT/Faults/f-control1/calc_f5 ==
  f-control : Inport
  f-s : Inport  Port=2
  Bus Selector : BusSelector  OutputSignals=EnF,IncipF,AutoF
  Bus Selector1 : BusSelector  OutputSignals=f5
  Constant : Constant  Value=p
  Product : Product  Inputs=3
  RAMP : simulink/Sources/Ramp  slope=amp/st  start=from  InitialOutput=0
  Saturation : Saturate  UpperLimit=abs(amp)  LowerLimit=-abs(amp)
  Step : Step  Time=from  After=amp  SampleTime=0
  Step1 : Step  Time=from+st  After=-amp  SampleTime=0
  Subsystem : Subsystem
  Sum : Sum  Inputs=|++
  Sum1 : Sum  Inputs=++|
  Switch:auto : Switch  Criteria=u2 > Threshold  Threshold=0.5  SaturateOnIntegerOverflow=off  InputSameDT=off
  Switch:kind : Switch  Criteria=u2 > Threshold  Threshold=0.5  SaturateOnIntegerOverflow=off  InputSameDT=off
  f : Outport  VectorParamsAs1DForOutWhenUnconnected=off
  wires:
  f-control/1 -> Bus Selector/1
  f-s/1 -> Bus Selector1/1
  Product/1 -> f/1
  Bus Selector/1 -> Product/1  "<EnF>"
  Bus Selector/2 -> Subsystem/1(IncipF), Switch:kind/2  "<IncipF>"
  Bus Selector/3 -> Switch:auto/2  "<AutoF>"
  Switch:auto/1 -> Product/2
  Sum/1 -> Switch:kind/1
  Sum1/1 -> Switch:kind/3
  Switch:kind/1 -> Switch:auto/1
  Step/1 -> Sum1/2
  Step1/1 -> Sum/2, Sum1/1
  Saturation/1 -> Sum/1
  RAMP/1 -> Saturation/1
  Constant/1 -> Product/3
  Bus Selector1/1 -> Subsystem/2(w)  "<f5>"
  Subsystem/1(w_sim) -> Switch:auto/3

== system TTS2_EXT/Faults/f-control1/calc_f51 ==
  f-control : Inport
  f-s : Inport  Port=2
  Bus Selector : BusSelector  OutputSignals=EnF,IncipF,AutoF
  Bus Selector1 : BusSelector  OutputSignals=f51
  Constant : Constant  Value=p
  Product : Product  Inputs=3
  RAMP : simulink/Sources/Ramp  slope=amp/st  start=from  InitialOutput=0
  Saturation : Saturate  UpperLimit=abs(amp)  LowerLimit=-abs(amp)
  Step : Step  Time=from  After=amp  SampleTime=0
  Step1 : Step  Time=from+st  After=-amp  SampleTime=0
  Subsystem : Subsystem
  Sum : Sum  Inputs=|++
  Sum1 : Sum  Inputs=++|
  Switch:auto : Switch  Criteria=u2 > Threshold  Threshold=0.5  SaturateOnIntegerOverflow=off  InputSameDT=off
  Switch:kind : Switch  Criteria=u2 > Threshold  Threshold=0.5  SaturateOnIntegerOverflow=off  InputSameDT=off
  f : Outport  VectorParamsAs1DForOutWhenUnconnected=off
  wires:
  f-control/1 -> Bus Selector/1
  f-s/1 -> Bus Selector1/1
  Product/1 -> f/1
  Bus Selector/1 -> Product/1  "<EnF>"
  Bus Selector/2 -> Subsystem/1(IncipF), Switch:kind/2  "<IncipF>"
  Bus Selector/3 -> Switch:auto/2  "<AutoF>"
  Switch:auto/1 -> Product/2
  Sum/1 -> Switch:kind/1
  Sum1/1 -> Switch:kind/3
  Switch:kind/1 -> Switch:auto/1
  Step/1 -> Sum1/2
  Step1/1 -> Sum/2, Sum1/1
  Saturation/1 -> Sum/1
  RAMP/1 -> Saturation/1
  Constant/1 -> Product/3
  Bus Selector1/1 -> Subsystem/2(w)  "<f51>"
  Subsystem/1(w_sim) -> Switch:auto/3

== system TTS2_EXT/Faults/f-control1/calc_f52 ==
  f-control : Inport
  f-s : Inport  Port=2
  Bus Selector : BusSelector  OutputSignals=EnF,IncipF,AutoF
  Bus Selector1 : BusSelector  OutputSignals=f52
  Constant : Constant  Value=p
  Product : Product  Inputs=3
  RAMP : simulink/Sources/Ramp  slope=amp/st  start=from  InitialOutput=0
  Saturation : Saturate  UpperLimit=abs(amp)  LowerLimit=-abs(amp)
  Step : Step  Time=from  After=amp  SampleTime=0
  Step1 : Step  Time=from+st  After=-amp  SampleTime=0
  Subsystem : Subsystem
  Sum : Sum  Inputs=|++
  Sum1 : Sum  Inputs=++|
  Switch:auto : Switch  Criteria=u2 > Threshold  Threshold=0.5  SaturateOnIntegerOverflow=off  InputSameDT=off
  Switch:kind : Switch  Criteria=u2 > Threshold  Threshold=0.5  SaturateOnIntegerOverflow=off  InputSameDT=off
  f : Outport  VectorParamsAs1DForOutWhenUnconnected=off
  wires:
  f-control/1 -> Bus Selector/1
  f-s/1 -> Bus Selector1/1
  Product/1 -> f/1
  Bus Selector/1 -> Product/1  "<EnF>"
  Bus Selector/2 -> Subsystem/1(IncipF), Switch:kind/2  "<IncipF>"
  Bus Selector/3 -> Switch:auto/2  "<AutoF>"
  Switch:auto/1 -> Product/2
  Sum/1 -> Switch:kind/1
  Sum1/1 -> Switch:kind/3
  Switch:kind/1 -> Switch:auto/1
  Step/1 -> Sum1/2
  Step1/1 -> Sum/2, Sum1/1
  Saturation/1 -> Sum/1
  RAMP/1 -> Saturation/1
  Constant/1 -> Product/3
  Bus Selector1/1 -> Subsystem/2(w)  "<f52>"
  Subsystem/1(w_sim) -> Switch:auto/3

== system TTS2_EXT/Faults/f-control1/calc_f53 ==
  f-control : Inport
  f-s : Inport  Port=2
  Bus Selector : BusSelector  OutputSignals=EnF,IncipF,AutoF
  Bus Selector1 : BusSelector  OutputSignals=f53
  Constant : Constant  Value=p
  Product : Product  Inputs=3
  RAMP : simulink/Sources/Ramp  slope=amp/st  start=from  InitialOutput=0
  Saturation : Saturate  UpperLimit=abs(amp)  LowerLimit=-abs(amp)
  Step : Step  Time=from  After=amp  SampleTime=0
  Step1 : Step  Time=from+st  After=-amp  SampleTime=0
  Subsystem : Subsystem
  Sum : Sum  Inputs=|++
  Sum1 : Sum  Inputs=++|
  Switch:auto : Switch  Criteria=u2 > Threshold  Threshold=0.5  SaturateOnIntegerOverflow=off  InputSameDT=off
  Switch:kind : Switch  Criteria=u2 > Threshold  Threshold=0.5  SaturateOnIntegerOverflow=off  InputSameDT=off
  f : Outport  VectorParamsAs1DForOutWhenUnconnected=off
  wires:
  f-control/1 -> Bus Selector/1
  f-s/1 -> Bus Selector1/1
  Product/1 -> f/1
  Bus Selector/1 -> Product/1  "<EnF>"
  Bus Selector/2 -> Subsystem/1(IncipF), Switch:kind/2  "<IncipF>"
  Bus Selector/3 -> Switch:auto/2  "<AutoF>"
  Switch:auto/1 -> Product/2
  Sum/1 -> Switch:kind/1
  Sum1/1 -> Switch:kind/3
  Switch:kind/1 -> Switch:auto/1
  Step/1 -> Sum1/2
  Step1/1 -> Sum/2, Sum1/1
  Saturation/1 -> Sum/1
  RAMP/1 -> Saturation/1
  Constant/1 -> Product/3
  Bus Selector1/1 -> Subsystem/2(w)  "<f53>"
  Subsystem/1(w_sim) -> Switch:auto/3

== system TTS2_EXT/Faults/f-control1/calc_f54 ==
  f-control : Inport
  f-s : Inport  Port=2
  Bus Selector : BusSelector  OutputSignals=EnF,IncipF,AutoF
  Bus Selector1 : BusSelector  OutputSignals=f54
  Constant : Constant  Value=p
  Product : Product  Inputs=3
  RAMP : simulink/Sources/Ramp  slope=amp/st  start=from  InitialOutput=0
  Saturation : Saturate  UpperLimit=abs(amp)  LowerLimit=-abs(amp)
  Step : Step  Time=from  After=amp  SampleTime=0
  Step1 : Step  Time=from+st  After=-amp  SampleTime=0
  Subsystem : Subsystem
  Sum : Sum  Inputs=|++
  Sum1 : Sum  Inputs=++|
  Switch:auto : Switch  Criteria=u2 > Threshold  Threshold=0.5  SaturateOnIntegerOverflow=off  InputSameDT=off
  Switch:kind : Switch  Criteria=u2 > Threshold  Threshold=0.5  SaturateOnIntegerOverflow=off  InputSameDT=off
  f : Outport  VectorParamsAs1DForOutWhenUnconnected=off
  wires:
  f-control/1 -> Bus Selector/1
  f-s/1 -> Bus Selector1/1
  Product/1 -> f/1
  Bus Selector/1 -> Product/1  "<EnF>"
  Bus Selector/2 -> Subsystem/1(IncipF), Switch:kind/2  "<IncipF>"
  Bus Selector/3 -> Switch:auto/2  "<AutoF>"
  Switch:auto/1 -> Product/2
  Sum/1 -> Switch:kind/1
  Sum1/1 -> Switch:kind/3
  Switch:kind/1 -> Switch:auto/1
  Step/1 -> Sum1/2
  Step1/1 -> Sum/2, Sum1/1
  Saturation/1 -> Sum/1
  RAMP/1 -> Saturation/1
  Constant/1 -> Product/3
  Bus Selector1/1 -> Subsystem/2(w)  "<f54>"
  Subsystem/1(w_sim) -> Switch:auto/3

== system TTS2_EXT/Faults/f-control1/calc_f55 ==
  f-control : Inport
  f-s : Inport  Port=2
  Bus Selector : BusSelector  OutputSignals=EnF,AutoF
  Bus Selector1 : BusSelector  OutputSignals=f55
  Constant : Constant  Value=p
  Product : Product  Inputs=3
  Step : Step  Time=from  After=amp  SampleTime=0
  Step1 : Step  Time=from+st  After=-amp  SampleTime=0
  Subsystem : Subsystem
  Sum1 : Sum  Inputs=++|
  Switch:auto : Switch  Criteria=u2 > Threshold  Threshold=0.5  SaturateOnIntegerOverflow=off  InputSameDT=off
  f : Outport  VectorParamsAs1DForOutWhenUnconnected=off
  wires:
  f-control/1 -> Bus Selector/1
  f-s/1 -> Bus Selector1/1
  Product/1 -> f/1
  Bus Selector/1 -> Product/1  "<EnF>"
  Bus Selector/2 -> Switch:auto/2  "<AutoF>"
  Switch:auto/1 -> Product/2
  Step/1 -> Sum1/2
  Step1/1 -> Sum1/1
  Constant/1 -> Product/3
  Bus Selector1/1 -> Subsystem/1(w)  "<f55>"
  Subsystem/1(w_sim) -> Switch:auto/3
  Sum1/1 -> Switch:auto/1

== system TTS2_EXT/Faults/f-control1/calc_f6 ==
  f-control : Inport
  f-s : Inport  Port=2
  Bus Selector : BusSelector  OutputSignals=EnF,IncipF,AutoF
  Bus Selector1 : BusSelector  OutputSignals=f6
  Constant : Constant  Value=p
  Product : Product  Inputs=3
  RAMP : simulink/Sources/Ramp  slope=amp/st  start=from  InitialOutput=0
  Saturation : Saturate  UpperLimit=abs(amp)  LowerLimit=-abs(amp)
  Step : Step  Time=from  After=amp  SampleTime=0
  Step1 : Step  Time=from+st  After=-amp  SampleTime=0
  Subsystem : Subsystem
  Sum : Sum  Inputs=|++
  Sum1 : Sum  Inputs=++|
  Switch:auto : Switch  Criteria=u2 > Threshold  Threshold=0.5  SaturateOnIntegerOverflow=off  InputSameDT=off
  Switch:kind : Switch  Criteria=u2 > Threshold  Threshold=0.5  SaturateOnIntegerOverflow=off  InputSameDT=off
  f : Outport  VectorParamsAs1DForOutWhenUnconnected=off
  wires:
  f-control/1 -> Bus Selector/1
  f-s/1 -> Bus Selector1/1
  Product/1 -> f/1
  Bus Selector/1 -> Product/1  "<EnF>"
  Bus Selector/2 -> Subsystem/1(IncipF), Switch:kind/2  "<IncipF>"
  Bus Selector/3 -> Switch:auto/2  "<AutoF>"
  Switch:auto/1 -> Product/2
  Sum/1 -> Switch:kind/1
  Sum1/1 -> Switch:kind/3
  Switch:kind/1 -> Switch:auto/1
  Step/1 -> Sum1/2
  Step1/1 -> Sum/2, Sum1/1
  Saturation/1 -> Sum/1
  RAMP/1 -> Saturation/1
  Constant/1 -> Product/3
  Bus Selector1/1 -> Subsystem/2(w)  "<f6>"
  Subsystem/1(w_sim) -> Switch:auto/3

== system TTS2_EXT/Faults/f-control1/calc_f7 ==
  f-control : Inport
  f-s : Inport  Port=2
  Bus Selector : BusSelector  OutputSignals=EnF,IncipF,AutoF
  Bus Selector1 : BusSelector  OutputSignals=f7
  Constant : Constant  Value=p
  Product : Product  Inputs=3
  RAMP : simulink/Sources/Ramp  slope=amp/st  start=from  InitialOutput=0
  Saturation : Saturate  UpperLimit=abs(amp)  LowerLimit=-abs(amp)
  Step : Step  Time=from  After=amp  SampleTime=0
  Step1 : Step  Time=from+st  After=-amp  SampleTime=0
  Subsystem : Subsystem
  Sum : Sum  Inputs=|++
  Sum1 : Sum  Inputs=++|
  Switch:auto : Switch  Criteria=u2 > Threshold  Threshold=0.5  SaturateOnIntegerOverflow=off  InputSameDT=off
  Switch:kind : Switch  Criteria=u2 > Threshold  Threshold=0.5  SaturateOnIntegerOverflow=off  InputSameDT=off
  f : Outport  VectorParamsAs1DForOutWhenUnconnected=off
  wires:
  f-control/1 -> Bus Selector/1
  f-s/1 -> Bus Selector1/1
  Product/1 -> f/1
  Bus Selector/1 -> Product/1  "<EnF>"
  Bus Selector/2 -> Subsystem/1(IncipF), Switch:kind/2  "<IncipF>"
  Bus Selector/3 -> Switch:auto/2  "<AutoF>"
  Switch:auto/1 -> Product/2
  Sum/1 -> Switch:kind/1
  Sum1/1 -> Switch:kind/3
  Switch:kind/1 -> Switch:auto/1
  Step/1 -> Sum1/2
  Step1/1 -> Sum/2, Sum1/1
  Saturation/1 -> Sum/1
  RAMP/1 -> Saturation/1
  Constant/1 -> Product/3
  Bus Selector1/1 -> Subsystem/2(w)  "<f7>"
  Subsystem/1(w_sim) -> Switch:auto/3

== system TTS2_EXT/Faults/f-control1/calc_f8 ==
  f-control : Inport
  f-s : Inport  Port=2
  Bus Selector : BusSelector  OutputSignals=EnF,IncipF,AutoF
  Bus Selector1 : BusSelector  OutputSignals=f8
  Constant : Constant  Value=p
  Product : Product  Inputs=3
  RAMP : simulink/Sources/Ramp  slope=amp/st  start=from  InitialOutput=0
  Saturation : Saturate  UpperLimit=abs(amp)  LowerLimit=-abs(amp)
  Step : Step  Time=from  After=amp  SampleTime=0
  Step1 : Step  Time=from+st  After=-amp  SampleTime=0
  Subsystem : Subsystem
  Sum : Sum  Inputs=|++
  Sum1 : Sum  Inputs=++|
  Switch:auto : Switch  Criteria=u2 > Threshold  Threshold=0.5  SaturateOnIntegerOverflow=off  InputSameDT=off
  Switch:kind : Switch  Criteria=u2 > Threshold  Threshold=0.5  SaturateOnIntegerOverflow=off  InputSameDT=off
  f : Outport  VectorParamsAs1DForOutWhenUnconnected=off
  wires:
  f-control/1 -> Bus Selector/1
  f-s/1 -> Bus Selector1/1
  Product/1 -> f/1
  Bus Selector/1 -> Product/1  "<EnF>"
  Bus Selector/2 -> Subsystem/1(IncipF), Switch:kind/2  "<IncipF>"
  Bus Selector/3 -> Switch:auto/2  "<AutoF>"
  Switch:auto/1 -> Product/2
  Sum/1 -> Switch:kind/1
  Sum1/1 -> Switch:kind/3
  Switch:kind/1 -> Switch:auto/1
  Step/1 -> Sum1/2
  Step1/1 -> Sum/2, Sum1/1
  Saturation/1 -> Sum/1
  RAMP/1 -> Saturation/1
  Constant/1 -> Product/3
  Bus Selector1/1 -> Subsystem/2(w)  "<f8>"
  Subsystem/1(w_sim) -> Switch:auto/3

== system TTS2_EXT/Faults/f-control1/calc_f9 ==
  f-control : Inport
  f-s : Inport  Port=2
  Bus Selector : BusSelector  OutputSignals=EnF,IncipF,AutoF
  Bus Selector1 : BusSelector  OutputSignals=f9
  Constant : Constant  Value=p
  Product : Product  Inputs=3
  RAMP : simulink/Sources/Ramp  slope=amp/st  start=from  InitialOutput=0
  Saturation : Saturate  UpperLimit=abs(amp)  LowerLimit=-abs(amp)
  Step : Step  Time=from  After=amp  SampleTime=0
  Step1 : Step  Time=from+st  After=-amp  SampleTime=0
  Subsystem : Subsystem
  Sum : Sum  Inputs=|++
  Sum1 : Sum  Inputs=++|
  Switch:auto : Switch  Criteria=u2 > Threshold  Threshold=0.5  SaturateOnIntegerOverflow=off  InputSameDT=off
  Switch:kind : Switch  Criteria=u2 > Threshold  Threshold=0.5  SaturateOnIntegerOverflow=off  InputSameDT=off
  f : Outport  VectorParamsAs1DForOutWhenUnconnected=off
  wires:
  f-control/1 -> Bus Selector/1
  f-s/1 -> Bus Selector1/1
  Product/1 -> f/1
  Bus Selector/1 -> Product/1  "<EnF>"
  Bus Selector/2 -> Subsystem/1(IncipF), Switch:kind/2  "<IncipF>"
  Bus Selector/3 -> Switch:auto/2  "<AutoF>"
  Switch:auto/1 -> Product/2
  Sum/1 -> Switch:kind/1
  Sum1/1 -> Switch:kind/3
  Switch:kind/1 -> Switch:auto/1
  Step/1 -> Sum1/2
  Step1/1 -> Sum/2, Sum1/1
  Saturation/1 -> Sum/1
  RAMP/1 -> Saturation/1
  Constant/1 -> Product/3
  Bus Selector1/1 -> Subsystem/2(w)  "<f9>"
  Subsystem/1(w_sim) -> Switch:auto/3
